simulink model "slmg1"  (Simulink 2.20)
settings: Solver=ode45  StartTime=0.0  StopTime=1200  MaxStep=0.1  RelTol=1e-3  AbsTol=1e-3
libraries: simulink x1
settings Model: SaveTime=off  SaveOutput=off  ConsistencyChecking=off  RTWPlaceOutputsASAP=off

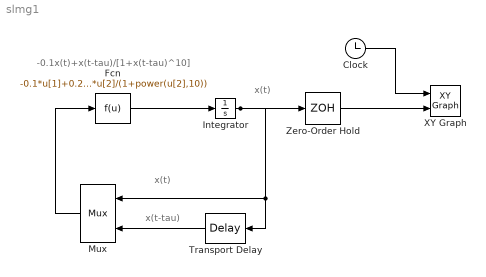
== system slmg1 ==
  note: x(t)
  note: x(t-tau)
  note: x(t)
  note: -0.1x(t)+x(t-tau)/[1+x(t-tau)^10]
  Clock : Clock
  Fcn : Fcn  Expr=-0.1*u[1]+0.2*u[2]/(1+power(u[2],10))
  Integrator : Integrator  ExternalReset=none  InitialConditionSource=internal  InitialCondition=1.2  LimitOutput=off  UpperSaturationLimit=inf  LowerSaturationLimit=-inf  ShowSaturationPort=off  ShowStatePort=off  AbsoluteTolerance=auto
  Mux : Mux  Orientation=left  Inputs=2
  Transport Delay : TransportDelay  Orientation=left  DelayTime=17  InitialInput=0  BufferSize=1024
  XY Graph : simulink/Sinks/XY Graph  xmin=0  xmax=1200  ymin=0.2  ymax=1.4  st=-1
  Zero-Order Hold : ZeroOrderHold  SampleTime=1
  wires:
  Fcn/1 -> Integrator/1
  Transport Delay/1 -> Mux/2
  Mux/1 -> Fcn/1
  Integrator/1 -> Zero-Order Hold/1, Transport Delay/1, Mux/1
  Zero-Order Hold/1 -> XY Graph/2
  Clock/1 -> XY Graph/1
